simulink model "kupf_sim"  (R2020b)
settings: Solver=VariableStepAuto  StartTime=0.0  StopTime=50  RelTol=1e-3
settings Model: Creator=mbober  LastModifiedBy=mbober

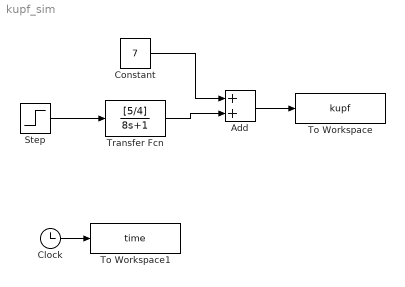
== system kupf_sim ==
  Add : Sum
  Clock : Clock
  Constant : Constant  Value=7
  Step : Step  Time=2  After=4  SampleTime=0
  To Workspace : ToWorkspace  VariableName=kupf  SampleTime=-1
  To Workspace1 : ToWorkspace  VariableName=time  SampleTime=-1
  Transfer Fcn : TransferFcn  Numerator=[5/4]  Denominator=[8 1]
  wires:
  Transfer Fcn/1 -> Add/2
  Constant/1 -> Add/1
  Add/1 -> To Workspace/1
  Step/1 -> Transfer Fcn/1
  Clock/1 -> To Workspace1/1
